simulink model "ON_OFF_LAZY"  (Simulink 7.7)
settings: Solver=ode3  StartTime=0.0  StopTime=10.0  FixedStep=5  RelTol=1e-3
settings Model: Creator=danwheeler  LastModifiedBy=danwheeler
settings DataIOCC: ExternalInput=UT  LoadExternalInput=on  SaveCompleteFinalSimState=on

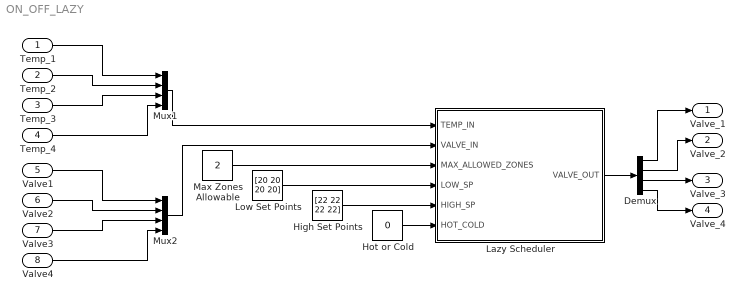
== system ON_OFF_LAZY ==
  Temp_1 : Inport
  Temp_2 : Inport  Port=2
  Temp_3 : Inport  Port=3
  Temp_4 : Inport  Port=4
  Valve1 : Inport  Port=5
  Valve2 : Inport  Port=6
  Valve3 : Inport  Port=7
  Valve4 : Inport  Port=8
  Demux : Demux
  High Set Points : Constant  Value=[22 22 22 22]
  Hot or Cold : Constant  Value=0
  Lazy Scheduler : Stateflow chart  TreatAsAtomicUnit=on
  Low Set Points : Constant  Value=[20 20 20 20]
  Max Zones Allowable : Constant  Value=2
  Mux1 : Mux
  Mux2 : Mux
  Valve_1 : Outport
  Valve_2 : Outport  Port=2
  Valve_3 : Outport  Port=3
  Valve_4 : Outport  Port=4
  wires:
  Temp_1/1 -> Mux1/1
  Temp_2/1 -> Mux1/2
  Temp_3/1 -> Mux1/3
  Temp_4/1 -> Mux1/4
  Mux1/1 -> Lazy Scheduler/1(TEMP_IN)
  Lazy Scheduler/1(VALVE_OUT) -> Demux/1
  Demux/1 -> Valve_1/1
  Demux/2 -> Valve_2/1
  Demux/3 -> Valve_3/1
  Demux/4 -> Valve_4/1
  Valve1/1 -> Mux2/1
  Valve2/1 -> Mux2/2
  Valve3/1 -> Mux2/3
  Valve4/1 -> Mux2/4
  Mux2/1 -> Lazy Scheduler/2(VALVE_IN)
  Max Zones Allowable/1 -> Lazy Scheduler/3(MAX_ALLOWED_ZONES)
  Low Set Points/1 -> Lazy Scheduler/4(LOW_SP)
  High Set Points/1 -> Lazy Scheduler/5(HIGH_SP)
  Hot or Cold/1 -> Lazy Scheduler/6(HOT_COLD)

== matlab function Lazy Scheduler ==
  data: TEMP_IN input double; VALVE_IN input double; MAX_ALLOWED_ZONES input double; LOW_SP input double; HIGH_SP input double; VALVE_OUT output double; HOT_COLD input double
function VALVE_OUT = fcn(TEMP_IN,VALVE_IN,MAX_ALLOWED_ZONES,LOW_SP,HIGH_SP,HOT_COLD)

CriticalStates = [0 0 0 0];
DesiredStates = [0 0 0 0];

VALVE_OUT = VALVE_IN;                                                      % Initialize output variable

% 
% COOLING
%
if HOT_COLD == 0
    %
    % TURN OFF ANY STATES THAT REACH LOW POINT
    %
    for i = 1:4
        if TEMP_IN(i) <= LOW_SP(i) && VALVE_IN(i) <= 90
            VALVE_OUT(i) = 90;
            VALVE_IN(i) = 90;   % Workaround for DETERMINE DESIRED STATES
        end 
    end

    %
    % FIND CRITICAL STATES, TURN THEM ALL ON
    %
    for i = 1:4
        if TEMP_IN(i) >= HIGH_SP(i)
            CriticalStates(i) = 1;
            VALVE_OUT(i) = 0;
        end    
    end
%
% HEATING
%
elseif HOT_COLD == 1
    %
    % TURN OFF ANY STATES THAT REACH HIGH POINT
    %
    for i = 1:4
        if TEMP_IN(i) >= HIGH_SP(i) && VALVE_IN(i) <= 90
            VALVE_OUT(i) = 90;
            VALVE_IN(i) = 90;   % Workaround for DETERMINE DESIRED STATES
        end 
    end

    %
    % FIND CRITICAL STATES, TURN THEM ALL ON
    %
    for i = 1:4
        if TEMP_IN(i) <= LOW_SP(i)
            CriticalStates(i) = 1;
            VALVE_OUT(i) = 0;
        end    
    end
end
DesiredStates( CriticalStates == 1 ) = 0;

%
% DETERMINE DESIRED STATES
%
for i = 1:4
    if VALVE_IN(i) < 90
        DesiredStates(i) = 1;
    end    
end

k = sum(CriticalStates);
m = sum(DesiredStates);

%
% HANDLE DESIRED STATES
%
if k >= MAX_ALLOWED_ZONES                                                  % If more or equal critical states are required as max allowed
    VALVE_OUT( DesiredStates == 1 ) = 90;
    VALVE_OUT( CriticalStates == 1 ) = 0;
else
    if m <= ( MAX_ALLOWED_ZONES - k )                                      % If we can leave them all on
        VALVE_OUT( DesiredStates == 1 ) = VALVE_IN( DesiredStates == 1);
    else                                                                   % We must pick some to turn off
        while k < MAX_ALLOWED_ZONES && sum( DesiredStates ) > 0
            des = find( DesiredStates == 1 );                              % Find the index of deisred states
            minVal = 1;                                                    % Randomly pick one
            maxVal = numel(des);                                           % ^
            randIndex = ceil(minVal + rand(1,1)*(maxVal-minVal));          % ^
            VALVE_OUT( des(randIndex) ) = 0;                               % Open the valve
            DesiredStates( des(randIndex) ) = 0;                           % Clear the desired state  
            k = k + 1;                                                     % Increment number of zones on
        end
        VALVE_OUT( DesiredStates == 1 )  = 90;                             % Close all desired states that did not make it through
    end
end
